simulink model "HalfWave_Rectifier"  (R2015a)
settings: Solver=ode23t  StartTime=0.0  StopTime=0.016*3.21  RelTol=1e-3
libraries: powerlib x10
settings Model: Creator=asus  LastModifiedBy=asus

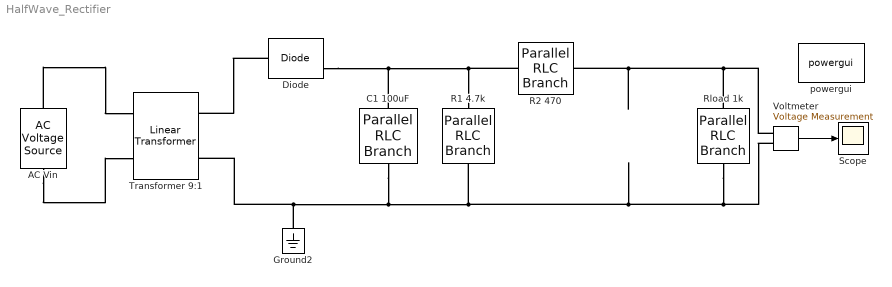
== system HalfWave_Rectifier ==
  " C1 100uF " : powerlib/Elements/Parallel RLC Branch  LConnTagsString=a  RConnTagsString=__new0  BranchType=C  Resistance=1  Inductance=1e-3  SetiL0=off  InitialCurrent=0  Capacitance=100e-6  Setx0=off  InitialVoltage=0  Measurements=None
  " Rload 1k   " : powerlib/Elements/Parallel RLC Branch  LConnTagsString=a  RConnTagsString=__new0  BranchType=R  Resistance=1000  Inductance=1e-3  SetiL0=off  InitialCurrent=0  Capacitance=1e-6  Setx0=off  InitialVoltage=0  Measurements=None
  " R2 470" : powerlib/Elements/Parallel RLC Branch  LConnTagsString=a  RConnTagsString=__new0  BranchType=R  Resistance=470  Inductance=1e-3  SetiL0=off  InitialCurrent=0  Capacitance=1e-6  Setx0=off  InitialVoltage=0  Measurements=None
  AC Vin : powerlib/Electrical Sources/AC Voltage Source  Amplitude=220*sqrt(2)  Phase=0  Frequency=60  SampleTime=0  Measurements=None
  Diode : powerlib/Power Electronics/Diode  Ron=0.001  Lon=0  Vf=0.8  IC=0  UseSnubber=off  Rs=0  Cs=0  Measurements=on
  Ground2 : powerlib/Elements/Ground  LConnTagsString=a
  R1 4.7k : powerlib/Elements/Parallel RLC Branch  LConnTagsString=a  RConnTagsString=__new0  BranchType=R  Resistance=4700  Inductance=1e-3  SetiL0=off  InitialCurrent=0  Capacitance=1e-6  Setx0=off  InitialVoltage=0  Measurements=None
  Scope : Scope
      settings: YMin=0  YMax=0.008
  Transformer 9:1 : powerlib/Elements/Linear Transformer  UNITS=SI  NominalPower=[ 250e6 60 ]  winding1=[220 0 0]  winding2=[24 0 0]  ThreeWindings=off  winding3=[12 0 0]  RmLm=[inf inf]  Measurements=None  DataType=on
  Voltmeter : powerlib/Measurements/Voltage Measurement  PhasorSimulation=off  OutputType=Complex  PSBequivalent=0
  powergui : powerlib/powergui  Priority=1  SimulationMode=Continuous  SolverType=Tustin/Backward Euler (TBE)  SampleTime=10e-6  frequency=60  SPID=on  DisableSnubberDevices=on  DisableRonSwitches=off  DisableVfSwitches=off  SwTol=0  DisplayEquations=off  Interpol=off  methode=off  Ts=100  FunctionMessages=off  echomessages=off  HookPort=off  EnableUseOfTLC=off  x0status=blocks  frequencyindice=60  Pbase=100e6  ErrMax=1e-4  Iterations=50  UnitsV=kV  UnitsW=MW  buscounter=0  RestoreLinks=warning  ResistiveCurrentMeasurement=off  Frange=[0:2:500]  Ylog=off  Xlog=on  ShowGrid=off  save=off  variable=ZData  structure=0  ZoomFFT=off  StartTime=0.0  cycles=1  DisplayStyle=1  fundamental=60  FreqAxis=off  MaxFrequency=1000  frequencyindicesteady=1  RmsSteady=1  display=off
  wires:
  Voltmeter/1 -> Scope/1
  connections:
  Diode/RConn1 -- " R2 470"/LConn1 -- R1 4.7k/LConn1 -- " C1 100uF "/LConn1
  Ground2/LConn1 -- Transformer 9:1/RConn2 -- " C1 100uF "/RConn1 -- " Rload 1k   "/RConn1 -- Voltmeter/LConn2 -- R1 4.7k/RConn1
  " Rload 1k   "/LConn1 -- Voltmeter/LConn1 -- " R2 470"/RConn1
  Diode/LConn1 -- Transformer 9:1/RConn1
  AC Vin/RConn1 -- Transformer 9:1/LConn1
  AC Vin/LConn1 -- Transformer 9:1/LConn2
